simulink model "Instalacion_Cascade"  (R2016b)
settings: Solver=ode23tb  StartTime=0.0  StopTime=2  RelTol=1e-3
libraries: powerlib x50, powerlib_meascontrol x12, simulink x8
settings Model: Creator=acasado  LastModifiedBy=acasado

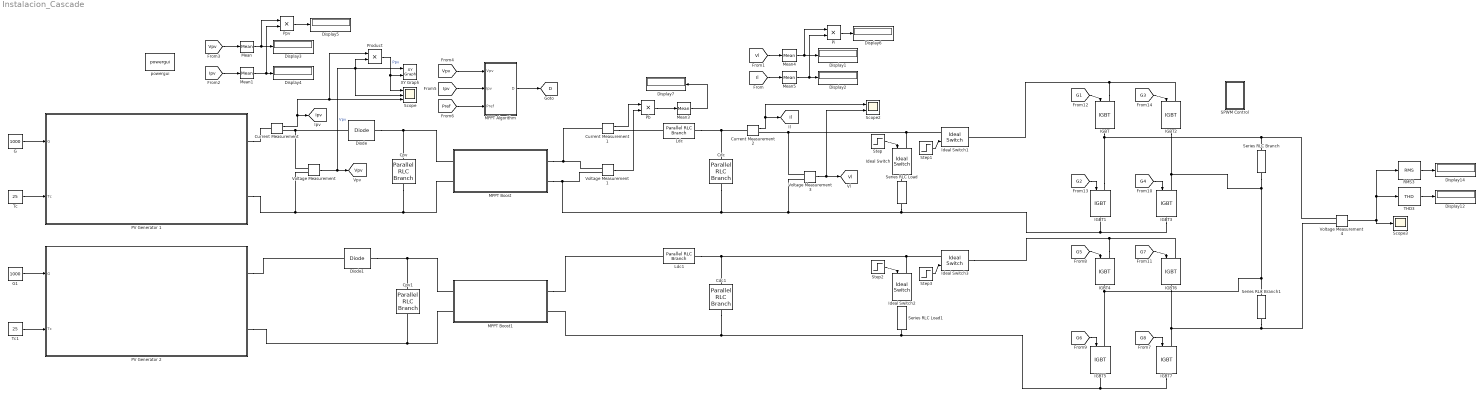
== system Instalacion_Cascade ==
  Cdc : powerlib/Elements/Parallel RLC Branch  LConnTagsString=a  RConnTagsString=__new0  BranchType=C  Resistance=1  Inductance=1e-3  SetiL0=off  InitialCurrent=0  Capacitance=4.7e-5  Setx0=off  InitialVoltage=20  Measurements=None
  Cdc1 : powerlib/Elements/Parallel RLC Branch  LConnTagsString=a  RConnTagsString=__new0  BranchType=C  Resistance=1  Inductance=1e-3  SetiL0=off  InitialCurrent=0  Capacitance=4.7e-5  Setx0=off  InitialVoltage=20  Measurements=None
  Cpv : powerlib/Elements/Parallel RLC Branch  LConnTagsString=a  RConnTagsString=__new0  BranchType=C  Resistance=1  Inductance=1e-3  SetiL0=off  InitialCurrent=0  Capacitance=4.7e-5  Setx0=off  InitialVoltage=0  Measurements=None
  Cpv1 : powerlib/Elements/Parallel RLC Branch  LConnTagsString=a  RConnTagsString=__new0  BranchType=C  Resistance=1  Inductance=1e-3  SetiL0=off  InitialCurrent=0  Capacitance=4.7e-5  Setx0=off  InitialVoltage=0  Measurements=None
  Current Measurement : powerlib/Measurements/Current Measurement  PhasorSimulation=off  OutputType=Complex  PSBequivalent=0
  Current Measurement1 : powerlib/Measurements/Current Measurement  PhasorSimulation=off  OutputType=Complex  PSBequivalent=0
  Current Measurement2 : powerlib/Measurements/Current Measurement  PhasorSimulation=off  OutputType=Complex  PSBequivalent=0
  Diode : powerlib/Power Electronics/Diode  Ron=0.001  Lon=0  Vf=0.8  IC=0  UseSnubber=off  Rs=500  Cs=250e-9  Measurements=off
  Diode1 : powerlib/Power Electronics/Diode  Ron=0.001  Lon=0  Vf=0.8  IC=0  UseSnubber=off  Rs=500  Cs=250e-9  Measurements=off
  Display{1..7,12,14} (9 alike) : Display
      Display5 settings: Decimation=2
      Display6 settings: Decimation=2
      Display7 settings: Decimation=2
  G : Constant  Value=1000
  G1 : Constant  Value=1000
  IGBT{,1..7} (8 alike) : powerlib/Power Electronics/IGBT  Ron=0.001  Lon=0  Vf=1  Tf=1e-6  Tt=2e-6  IC=0  Rs=1e5  Cs=inf  Measurements=off
  Ideal Switch{,1..3} (4 alike) : powerlib/Power Electronics/Ideal Switch  Ron=0.001  Lon=0  IC=0  Rs=1e5  Cs=inf  Measurements=off
  Ldc : powerlib/Elements/Parallel RLC Branch  LConnTagsString=a  RConnTagsString=__new0  BranchType=L  Resistance=1  Inductance=1e-3  SetiL0=off  InitialCurrent=0  Capacitance=1e-6  Setx0=off  InitialVoltage=0  Measurements=None
  Ldc1 : powerlib/Elements/Parallel RLC Branch  LConnTagsString=a  RConnTagsString=__new0  BranchType=L  Resistance=1  Inductance=1e-3  SetiL0=off  InitialCurrent=0  Capacitance=1e-6  Setx0=off  InitialVoltage=0  Measurements=None
  MPPT Algorithm : Subsystem  mask{N=3}
      mask TypeOptions N: 1 | 2 | 3 | 4
  MPPT Boost : Subsystem
      mask Display: image('\\Boole\Proyectos\LI_ROW_2017_SOLAR\BOOST.png')
  MPPT Boost1 : Subsystem
      mask Display: image('\\Boole\Proyectos\LI_ROW_2017_SOLAR\BOOST.png')
  Mean{,1,3..5} (5 alike) : powerlib_meascontrol/Measurements/Mean  Freq=10000  Vinit=0  Ts=0
  PV Generator 1 : Subsystem  mask{G=1000, Tc=25, Pmax=200, Isc=8.21, Voc=32.9, ki=3.18e-3/8.21, kv=-0.123/32.9, Ncs=54, n=1.3417, Rs=0.2172, Rsh=951.9317, Ns=3, Np=3}
      mask prompts: G "G (W/m2)"; Tc "Tc (ºC)"; Pmax "Pmax (W)"; Isc "Isc (A)"; Voc "Voc (V)"; ki "ki (%/º)"; kv "kv (%/º)"; Rs "Rs (ohm)"; Rsh "Rsh (ohm)"
      mask Display: image('\\Boole\Proyectos\LI_ROW_2017_SOLAR\string.jpg')
  PV Generator 2 : Subsystem  mask{G=1000, Tc=25, Pmax=200, Isc=8.21, Voc=32.9, ki=3.18e-3/8.21, kv=-0.123/32.9, Ncs=54, n=1.3417, Rs=0.2172, Rsh=951.9317, Ns=3, Np=3}
      mask prompts: G "G (W/m2)"; Tc "Tc (ºC)"; Pmax "Pmax (W)"; Isc "Isc (A)"; Voc "Voc (V)"; ki "ki (%/º)"; kv "kv (%/º)"; Rs "Rs (ohm)"; Rsh "Rsh (ohm)"
      mask Display: image('\\Boole\Proyectos\LI_ROW_2017_SOLAR\string.jpg')
  Pb : Product
  Pi : Product
  Ppv : Product
  Product : Product
  RMS3 : powerlib_meascontrol/Measurements/RMS  TrueRMS=on  Freq=50  RMSInit=0  Ts=0
  SPWM Control : Subsystem  mask{A=2, fm=3000, fs=50}
  Scope : Scope  NumInputPorts=3
  Scope2 : Scope  NumInputPorts=2
  Scope3 : Scope
  Series RLC Branch : powerlib/Elements/Series RLC Branch  LConnTagsString=__new0  RConnTagsString=__new0  BranchType=R  Resistance=100  Inductance=1e-3  SetiL0=off  InitialCurrent=0  Capacitance=1e-6  Setx0=off  InitialVoltage=0  Measurements=None
  Series RLC Branch1 : powerlib/Elements/Series RLC Branch  LConnTagsString=__new0  RConnTagsString=__new0  BranchType=R  Resistance=100  Inductance=1e-3  SetiL0=off  InitialCurrent=0  Capacitance=1e-6  Setx0=off  InitialVoltage=0  Measurements=None
  Series RLC Load : powerlib/Elements/Series RLC Load  LConnTagsString=a  RConnTagsString=__new0  NominalVoltage=100  NominalFrequency=10000  ActivePower=1000  InductivePower=0  CapacitivePower=0  Setx0=off  InitialVoltage=0  SetiL0=off  InitialCurrent=0  Measurements=None  LoadType=constant Z
  Series RLC Load1 : powerlib/Elements/Series RLC Load  LConnTagsString=a  RConnTagsString=__new0  NominalVoltage=100  NominalFrequency=10000  ActivePower=1000  InductivePower=0  CapacitivePower=0  Setx0=off  InitialVoltage=0  SetiL0=off  InitialCurrent=0  Measurements=None  LoadType=constant Z
  Step : Step  Time=0.02  Before=1  After=0  SampleTime=0
  Step1 : Step  Time=0.02  SampleTime=0
  Step2 : Step  Time=0.02  Before=1  After=0  SampleTime=0
  Step3 : Step  Time=0.02  SampleTime=0
  THD3 : powerlib_meascontrol/Measurements/THD  Freq=50  Ts=0
  Tc : Constant  Value=25
  Tc1 : Constant  Value=25
  Voltage Measurement{,1,3..4} (4 alike) : powerlib/Measurements/Voltage Measurement  PhasorSimulation=off  OutputType=Complex  PSBequivalent=0
  XY Graph : simulink/Sinks/XY Graph  xmin=0  xmax=33  ymin=0  ymax=205  st=-1
  powergui : powerlib/powergui  Priority=1  SimulationMode=Continuous  SolverType=Tustin/Backward Euler (TBE)  SampleTime=50e-6  frequency=60  SPID=off  DisableSnubberDevices=off  DisableRonSwitches=off  DisableVfSwitches=off  SwTol=0  DisplayEquations=off  Interpol=off  ExternalGateDelay=off  methode=off  Ts=10  FunctionMessages=off  echomessages=off  HookPort=off  EnableUseOfTLC=off  x0status=blocks  frequencyindice=0  Pbase=100e6  ErrMax=1e-4  Iterations=50  UnitsV=kV  UnitsW=MW  buscounter=0  RestoreLinks=warning  ResistiveCurrentMeasurement=off  Frange=[0:2:500]  Ylog=off  Xlog=on  ShowGrid=off  save=off  variable=ZData  structure=Bridge  ZoomFFT=on  StartTime=0.2  cycles=5  DisplayStyle=1  fundamental=50  FreqAxis=off  MaxFrequency=1000  frequencyindicesteady=1  RmsSteady=1  display=off
  tag scope: D=global, Il=global, Ipv=global, Vl=global, Vpv=global
  wires:
  Current Measurement/1 -> [Ipv], Scope/3, Product/1
  Voltage Measurement/1 -> [Vpv], Product/2, XY Graph/1, Scope/2  "Vpv"
  Voltage Measurement3/1 -> Scope2/2, [Vl]
  Current Measurement2/1 -> [Il], Scope2/1
  [Vpv] -> Mean/1
  [Ipv] -> Mean1/1
  Mean/1 -> Ppv/1, Display3/1
  Mean1/1 -> Ppv/2, Display4/1
  Product/1 -> Scope/1, XY Graph/2  "Ppv"
  Ppv/1 -> Display5/1
  Voltage Measurement1/1 -> Pb/2
  Current Measurement1/1 -> Pb/1
  Pb/1 -> Mean3/1
  Mean3/1 -> Display7/1
  [Vpv] -> MPPT Algorithm/1(Vpv)
  [Ipv] -> MPPT Algorithm/2(Ipv)
  MPPT Algorithm/1(D) -> [D]
  [Pref] -> MPPT Algorithm/3(Pref)
  [Vl] -> Mean4/1
  Mean4/1 -> Pi/1, Display1/1
  [Il] -> Mean5/1
  Mean5/1 -> Pi/2, Display2/1
  Pi/1 -> Display6/1
  Step/1 -> Ideal Switch/1
  Step1/1 -> Ideal Switch1/1
  G/1 -> PV Generator 1/1(G)
  Tc/1 -> PV Generator 1/2(Tc)
  Voltage Measurement4/1 -> RMS3/1, THD3/1, Scope3/1
  RMS3/1 -> Display14/1
  THD3/1 -> Display12/1
  Step2/1 -> Ideal Switch2/1
  Step3/1 -> Ideal Switch3/1
  [G1] -> IGBT/1
  [G3] -> IGBT2/1
  [G4] -> IGBT3/1
  [G2] -> IGBT1/1
  [G5] -> IGBT4/1
  [G7] -> IGBT6/1
  [G8] -> IGBT7/1
  [G6] -> IGBT5/1
  G1/1 -> PV Generator 2/1(G)
  Tc1/1 -> PV Generator 2/2(Tc)
  connections:
  Voltage Measurement/LConn1 -- Diode/LConn1 -- Current Measurement/RConn1
  Current Measurement1/LConn1 -- Voltage Measurement1/LConn1 -- MPPT Boost/RConn1
  Cdc/LConn1 -- Ldc/RConn1 -- Current Measurement2/LConn1
  Current Measurement1/RConn1 -- Ldc/LConn1
  Cpv/RConn1 -- MPPT Boost/LConn2 -- PV Generator 1/RConn2 -- Voltage Measurement/LConn2
  PV Generator 1/RConn1 -- Current Measurement/LConn1
  Voltage Measurement3/LConn1 -- Ideal Switch/LConn1 -- Ideal Switch1/LConn1 -- Current Measurement2/RConn1
  Ideal Switch/RConn1 -- Series RLC Load/LConn1
  IGBT/LConn1 -- Ideal Switch1/RConn1 -- IGBT2/LConn1
  Cpv/LConn1 -- Diode/RConn1 -- MPPT Boost/LConn1
  IGBT1/LConn1 -- Voltage Measurement4/LConn1 -- Series RLC Branch/LConn1 -- IGBT/RConn1
  IGBT2/RConn1 -- IGBT3/LConn1 -- IGBT5/LConn1 -- IGBT4/RConn1 -- Series RLC Branch1/LConn1 -- Series RLC Branch/RConn1
  MPPT Boost1/RConn1 -- Ldc1/LConn1
  Ldc1/RConn1 -- Cdc1/LConn1 -- Ideal Switch2/LConn1 -- Ideal Switch3/LConn1
  Cdc1/RConn1 -- Series RLC Load1/RConn1 -- IGBT7/RConn1 -- IGBT5/RConn1 -- MPPT Boost1/RConn2
  Series RLC Branch1/RConn1 -- IGBT6/RConn1 -- IGBT7/LConn1 -- Voltage Measurement4/LConn2
  IGBT4/LConn1 -- Ideal Switch3/RConn1 -- IGBT6/LConn1
  Voltage Measurement1/LConn2 -- MPPT Boost/RConn2 -- IGBT3/RConn1 -- IGBT1/RConn1 -- Series RLC Load/RConn1 -- Voltage Measurement3/LConn2 -- Cdc/RConn1
  PV Generator 2/RConn1 -- Diode1/LConn1
  Diode1/RConn1 -- Cpv1/LConn1 -- MPPT Boost1/LConn1
  MPPT Boost1/LConn2 -- Cpv1/RConn1 -- PV Generator 2/RConn2

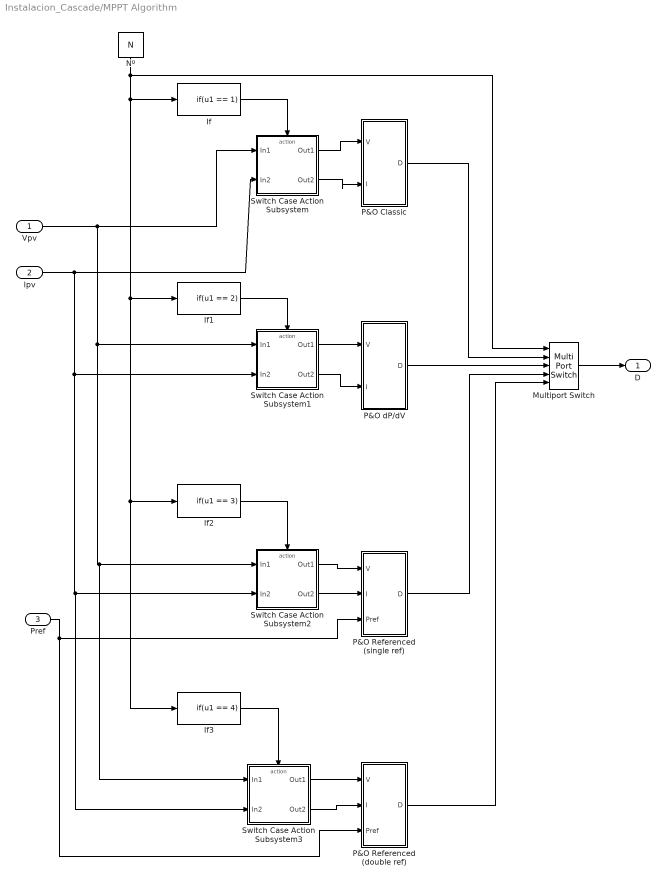
== system Instalacion_Cascade/MPPT Algorithm ==
  Vpv : Inport
  Ipv : Inport  Port=2
  Pref : Inport  Port=3
  If : If  IfExpression=u1 == 1  ShowElse=off
  If1 : If  IfExpression=u1 == 2  ShowElse=off
  If2 : If  IfExpression=u1 == 3  ShowElse=off
  If3 : If  IfExpression=u1 == 4  ShowElse=off
  Multiport Switch : MultiPortSwitch  DataPortOrder=Specify indices  DataPortIndices={1,2,3,4}
  Nº : Constant  Value=N
  P&O Classic : Subsystem
  P&O Referenced (double ref) : Subsystem
  P&O Referenced (single ref) : Subsystem
  P&O dP/dV : Subsystem
  Switch Case Action Subsystem : Subsystem  TreatAsAtomicUnit=on
  Switch Case Action Subsystem1 : Subsystem  TreatAsAtomicUnit=on
  Switch Case Action Subsystem2 : Subsystem  TreatAsAtomicUnit=on
  Switch Case Action Subsystem3 : Subsystem  TreatAsAtomicUnit=on
  D : Outport
  wires:
  Multiport Switch/1 -> D/1
  Pref/1 -> P&O Referenced (single ref)/3(Pref), P&O Referenced (double ref)/3(Pref)
  P&O Classic/1(D) -> Multiport Switch/2
  P&O dP/dV/1(D) -> Multiport Switch/3
  P&O Referenced (single ref)/1(D) -> Multiport Switch/4
  Nº/1 -> Multiport Switch/1, If/1, If3/1, If2/1, If1/1
  Switch Case Action Subsystem/2(Out2) -> P&O Classic/2(I)
  Switch Case Action Subsystem/1(Out1) -> P&O Classic/1(V)
  Switch Case Action Subsystem1/1(Out1) -> P&O dP/dV/1(V)
  Switch Case Action Subsystem1/2(Out2) -> P&O dP/dV/2(I)
  Switch Case Action Subsystem2/2(Out2) -> P&O Referenced (single ref)/2(I)
  Switch Case Action Subsystem2/1(Out1) -> P&O Referenced (single ref)/1(V)
  Vpv/1 -> Switch Case Action Subsystem3/1(In1), Switch Case Action Subsystem2/1(In1), Switch Case Action Subsystem1/1(In1), Switch Case Action Subsystem/1(In1)
  Ipv/1 -> Switch Case Action Subsystem3/2(In2), Switch Case Action Subsystem2/2(In2), Switch Case Action Subsystem1/2(In2), Switch Case Action Subsystem/2(In2)
  If1/1 -> Switch Case Action Subsystem1/Action
  If2/1 -> Switch Case Action Subsystem2/Action
  If/1 -> Switch Case Action Subsystem/Action
  P&O Referenced (double ref)/1(D) -> Multiport Switch/5
  Switch Case Action Subsystem3/1(Out1) -> P&O Referenced (double ref)/1(V)
  Switch Case Action Subsystem3/2(Out2) -> P&O Referenced (double ref)/2(I)
  If3/1 -> Switch Case Action Subsystem3/Action

== system Instalacion_Cascade/MPPT Boost ==
  C : powerlib/Elements/Parallel RLC Branch  LConnTagsString=a  RConnTagsString=__new0  BranchType=C  Resistance=1  Inductance=1e-3  SetiL0=off  InitialCurrent=0  Capacitance=3.2e-4  Setx0=off  InitialVoltage=20  Measurements=None
  Diode : powerlib/Power Electronics/Diode  Ron=0.001  Lon=0  Vf=0.8  IC=0  UseSnubber=off  Rs=500  Cs=250e-9  Measurements=off
  L : powerlib/Elements/Parallel RLC Branch  LConnTagsString=a  RConnTagsString=__new0  BranchType=L  Resistance=1  Inductance=1e-3  SetiL0=off  InitialCurrent=0  Capacitance=1e-6  Setx0=off  InitialVoltage=0  Measurements=None
  Mosfet : powerlib/Power Electronics/Mosfet  Ron=0.1  Lon=0  Rd=0.01  Vfd=0  IC=0  Rs=1e5  Cs=inf  Measurements=off
  Conn1 : PMIOPort  Port=1  Side=Left
  Conn3 : PMIOPort  Port=2  Side=Left
  Conn2 : PMIOPort  Port=3  Side=Right
  Conn4 : PMIOPort  Port=4  Side=Right
  wires:
  [D] -> Mosfet/1
  connections:
  Diode/RConn1 -- C/LConn1 -- Conn2/RConn1
  L/LConn1 -- Conn1/RConn1
  Mosfet/LConn1 -- Diode/LConn1 -- L/RConn1
  C/RConn1 -- Conn4/RConn1 -- Conn3/RConn1 -- Mosfet/RConn1

== system Instalacion_Cascade/MPPT Boost1 ==
  C : powerlib/Elements/Parallel RLC Branch  LConnTagsString=a  RConnTagsString=__new0  BranchType=C  Resistance=1  Inductance=1e-3  SetiL0=off  InitialCurrent=0  Capacitance=3.2e-4  Setx0=off  InitialVoltage=20  Measurements=None
  Diode : powerlib/Power Electronics/Diode  Ron=0.001  Lon=0  Vf=0.8  IC=0  UseSnubber=off  Rs=500  Cs=250e-9  Measurements=off
  L : powerlib/Elements/Parallel RLC Branch  LConnTagsString=a  RConnTagsString=__new0  BranchType=L  Resistance=1  Inductance=1e-3  SetiL0=off  InitialCurrent=0  Capacitance=1e-6  Setx0=off  InitialVoltage=0  Measurements=None
  Mosfet : powerlib/Power Electronics/Mosfet  Ron=0.1  Lon=0  Rd=0.01  Vfd=0  IC=0  Rs=1e5  Cs=inf  Measurements=off
  Conn1 : PMIOPort  Port=1  Side=Left
  Conn3 : PMIOPort  Port=2  Side=Left
  Conn2 : PMIOPort  Port=3  Side=Right
  Conn4 : PMIOPort  Port=4  Side=Right
  wires:
  [D] -> Mosfet/1
  connections:
  Mosfet/RConn1 -- Conn3/RConn1 -- Conn4/RConn1 -- C/RConn1
  L/RConn1 -- Diode/LConn1 -- Mosfet/LConn1
  L/LConn1 -- Conn1/RConn1
  Conn2/RConn1 -- C/LConn1 -- Diode/RConn1

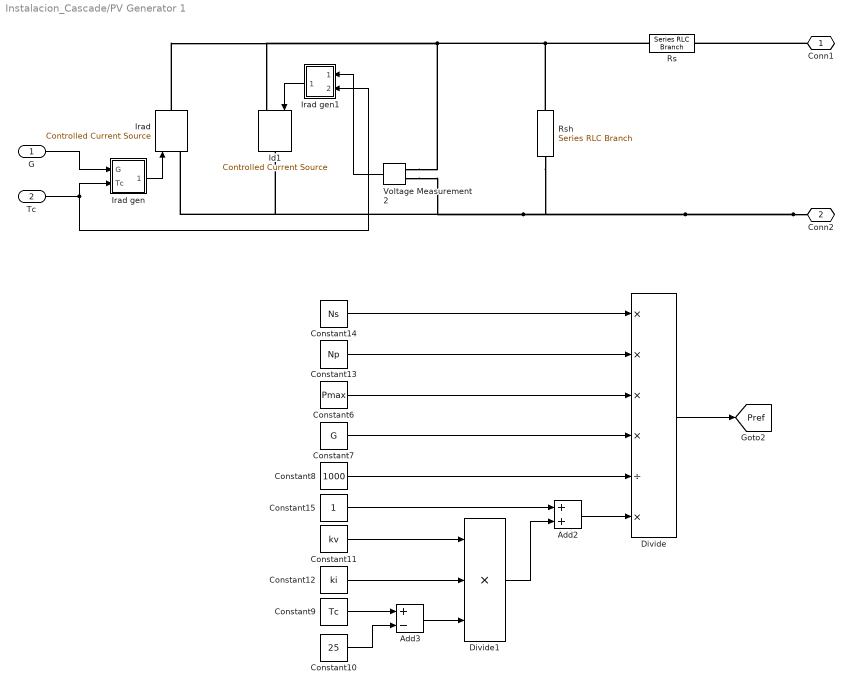
== system Instalacion_Cascade/PV Generator 1 ==
  G : Inport
  Tc : Inport  Port=2
  Add2 : Sum
  Add3 : Sum  Inputs=+-
  Constant10 : Constant  Value=25
  Constant11 : Constant  Value=kv
  Constant12 : Constant  Value=ki
  Constant13 : Constant  Value=Np
  Constant14 : Constant  Value=Ns
  Constant15 : Constant
  Constant6 : Constant  Value=Pmax
  Constant7 : Constant  Value=G
  Constant8 : Constant  Value=1000
  Constant9 : Constant  Value=Tc
  Divide : Product  Inputs=****/*
  Divide1 : Product  Inputs=***
  Id1 : powerlib/Electrical Sources/Controlled Current Source  Initialize=on  Source_Type=DC  Amplitude=0  Phase=0  Frequency=0  Measurements=None
  Irad : powerlib/Electrical Sources/Controlled Current Source  Initialize=off  Source_Type=DC  Amplitude=1  Phase=0  Frequency=0  Measurements=None
  Irad gen : Subsystem  mask{G=G, Tc=Tc, Isc=Isc, ki=ki, Np=Np}
  Irad gen1 : Subsystem  mask{n=n, Isc=Isc, Voc=Voc, ki=ki*Isc, kv=kv*Voc, Tc=Tc, Ncs=Ncs, Ns=Ns, Np=Np}
  Rs : powerlib/Elements/Series RLC Branch  LConnTagsString=__new0  RConnTagsString=__new0  BranchType=R  Resistance=Rs*Ns/Np  Inductance=1e-3  SetiL0=off  InitialCurrent=0  Capacitance=1e-6  Setx0=off  InitialVoltage=0  Measurements=None
  Rsh : powerlib/Elements/Series RLC Branch  LConnTagsString=__new0  RConnTagsString=__new0  BranchType=R  Resistance=Rsh*Ns/Np  Inductance=1e-3  SetiL0=off  InitialCurrent=0  Capacitance=1e-6  Setx0=off  InitialVoltage=0  Measurements=None
  Voltage Measurement2 : powerlib/Measurements/Voltage Measurement  PhasorSimulation=off  OutputType=Complex  PSBequivalent=0
  Conn1 : PMIOPort  Port=1  Side=Right
  Conn2 : PMIOPort  Port=2  Side=Right
  tag scope: Pref=global
  wires:
  Irad gen1/1(Id) -> Id1/1
  Voltage Measurement2/1 -> Irad gen1/1(Vd)
  Irad gen/1(Irad) -> Irad/1
  G/1 -> Irad gen/1(G)
  Tc/1 -> Irad gen1/2(Tc), Irad gen/2(Tc)
  Constant14/1 -> Divide/1
  Constant13/1 -> Divide/2
  Constant6/1 -> Divide/3
  Constant7/1 -> Divide/4
  Constant8/1 -> Divide/5
  Constant15/1 -> Add2/1
  Add2/1 -> Divide/6
  Divide1/1 -> Add2/2
  Constant9/1 -> Add3/1
  Constant10/1 -> Add3/2
  Add3/1 -> Divide1/3
  Constant11/1 -> Divide1/1
  Constant12/1 -> Divide1/2
  Divide/1 -> [Pref]
  connections:
  Conn2/RConn1 -- Id1/RConn1 -- Irad/LConn1 -- Voltage Measurement2/LConn2 -- Rsh/RConn1
  Rsh/LConn1 -- Rs/LConn1 -- Voltage Measurement2/LConn1 -- Id1/LConn1 -- Irad/RConn1
  Conn1/RConn1 -- Rs/RConn1

== system Instalacion_Cascade/PV Generator 2 ==
  G : Inport
  Tc : Inport  Port=2
  Id1 : powerlib/Electrical Sources/Controlled Current Source  Initialize=on  Source_Type=DC  Amplitude=0  Phase=0  Frequency=0  Measurements=None
  Irad : powerlib/Electrical Sources/Controlled Current Source  Initialize=off  Source_Type=DC  Amplitude=1  Phase=0  Frequency=0  Measurements=None
  Irad gen : Subsystem  mask{G=G, Tc=Tc, Isc=Isc, ki=ki, Np=Np}
  Irad gen1 : Subsystem  mask{n=n, Isc=Isc, Voc=Voc, ki=ki*Isc, kv=kv*Voc, Tc=Tc, Ncs=Ncs, Ns=Ns, Np=Np}
  Rs : powerlib/Elements/Series RLC Branch  LConnTagsString=__new0  RConnTagsString=__new0  BranchType=R  Resistance=Rs*Ns/Np  Inductance=1e-3  SetiL0=off  InitialCurrent=0  Capacitance=1e-6  Setx0=off  InitialVoltage=0  Measurements=None
  Rsh : powerlib/Elements/Series RLC Branch  LConnTagsString=__new0  RConnTagsString=__new0  BranchType=R  Resistance=Rsh*Ns/Np  Inductance=1e-3  SetiL0=off  InitialCurrent=0  Capacitance=1e-6  Setx0=off  InitialVoltage=0  Measurements=None
  Voltage Measurement2 : powerlib/Measurements/Voltage Measurement  PhasorSimulation=off  OutputType=Complex  PSBequivalent=0
  Conn1 : PMIOPort  Port=1  Side=Right
  Conn2 : PMIOPort  Port=2  Side=Right
  wires:
  Tc/1 -> Irad gen/2(Tc), Irad gen1/2(Tc)
  G/1 -> Irad gen/1(G)
  Irad gen/1(Irad) -> Irad/1
  Voltage Measurement2/1 -> Irad gen1/1(Vd)
  Irad gen1/1(Id) -> Id1/1
  connections:
  Conn1/RConn1 -- Rs/RConn1
  Irad/RConn1 -- Id1/LConn1 -- Voltage Measurement2/LConn1 -- Rs/LConn1 -- Rsh/LConn1
  Rsh/RConn1 -- Voltage Measurement2/LConn2 -- Irad/LConn1 -- Id1/RConn1 -- Conn2/RConn1

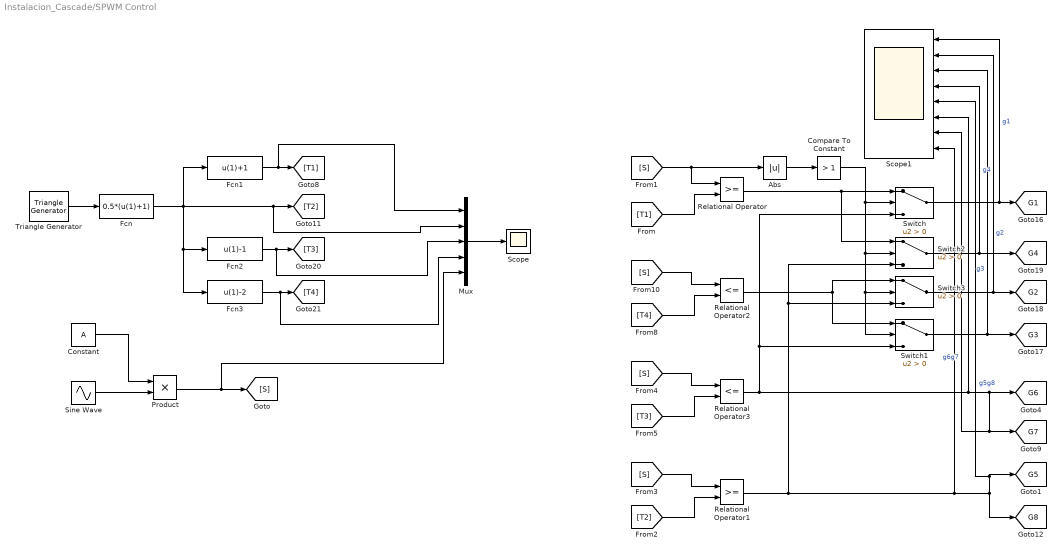
== system Instalacion_Cascade/SPWM Control ==
  Abs : Abs
  Compare To Constant : simulink/Logic and Bit Operations/Compare To Constant  relop=>  const=1  OutDataTypeStr=boolean
  Constant : Constant  Value=A
  Fcn : Fcn  Expr=0.5*(u(1)+1)
  Fcn1 : Fcn  Expr=u(1)+1
  Fcn2 : Fcn  Expr=u(1)-1
  Fcn3 : Fcn  Expr=u(1)-2
  Mux : Mux  Inputs=5
  Product : Product
  Relational Operator : RelationalOperator  OutDataTypeStr=boolean  RndMeth=Simplest
  Relational Operator1 : RelationalOperator  OutDataTypeStr=boolean  RndMeth=Simplest
  Relational Operator2 : RelationalOperator  Operator=<=  OutDataTypeStr=boolean  RndMeth=Simplest
  Relational Operator3 : RelationalOperator  Operator=<=  OutDataTypeStr=boolean  RndMeth=Simplest
  Scope : Scope
  Scope1 : Scope  NumInputPorts=8
  Sine Wave : Sin  Frequency=fs*2*pi  SampleTime=0
  Switch{,1..3} (4 alike) : Switch  Criteria=u2 > Threshold
  Triangle Generator : powerlib_meascontrol/Pulse & Signal Generators/Triangle Generator  Freq=fm  Phase=90  Ts=0
  tag scope: G1=global, G2=global, G3=global, G4=global, G5=global, G6=global, G7=global, G8=global
  wires:
  Sine Wave/1 -> Product/2
  Constant/1 -> Product/1
  Product/1 -> Mux/5, [S]
  Fcn/1 -> Mux/2, [T2], Fcn2/1, Fcn3/1, Fcn1/1
  Fcn1/1 -> Mux/1, [T1]
  Fcn2/1 -> Mux/3, [T3]
  Fcn3/1 -> Mux/4, [T4]
  Triangle Generator/1 -> Fcn/1
  Mux/1 -> Scope/1
  [S] -> Abs/1, Relational Operator/1
  [T1] -> Relational Operator/2
  [S] -> Relational Operator2/1
  [T4] -> Relational Operator2/2
  [S] -> Relational Operator1/1
  [T2] -> Relational Operator1/2
  [S] -> Relational Operator3/1
  [T3] -> Relational Operator3/2
  Switch/1 -> Scope1/1, [G1]  "g1"
  Relational Operator/1 -> Switch2/1, Switch/1
  Abs/1 -> Compare To Constant/1
  Compare To Constant/1 -> Switch2/2, Switch3/2, Switch1/2, Switch/2
  Relational Operator1/1 -> Switch3/3, Switch2/3, Scope1/8, Scope1/5, [G5], [G8]  "g5g8"
  Switch1/1 -> Scope1/3, [G3]  "g3"
  Relational Operator2/1 -> Switch3/1, Switch1/1
  Relational Operator3/1 -> Switch1/3, Switch/3, Scope1/6, Scope1/7, [G7], [G6]  "g6g7"
  Switch2/1 -> Scope1/4, [G4]  "g4"
  Switch3/1 -> Scope1/2, [G2]  "g2"

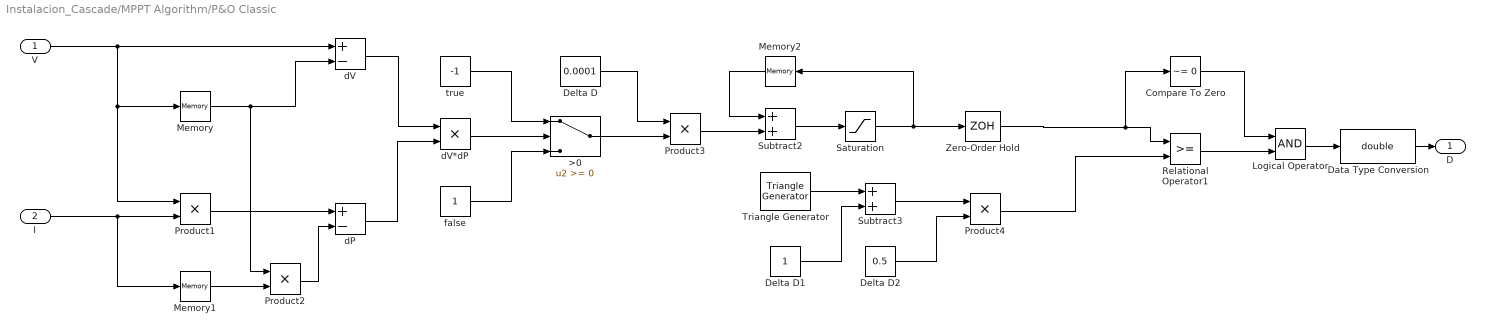
== system Instalacion_Cascade/MPPT Algorithm/P&O Classic ==
  V : Inport
  I : Inport  Port=2
  >0 : Switch  ZeroCross=off
  Compare To Zero : simulink/Logic and Bit Operations/Compare To Zero  relop=~=  OutDataTypeStr=boolean
  Data Type Conversion : DataTypeConversion  OutDataTypeStr=double
  Delta D : Constant  Value=0.0001
  Delta D1 : Constant
  Delta D2 : Constant  Value=0.5
  Logical Operator : Logic  AllPortsSameDT=off  OutDataTypeStr=boolean
  Memory : Memory
  Memory1 : Memory  X0=8.21
  Memory2 : Memory  X0=0.5
  Product{1..4} (4 alike) : Product
  Relational Operator1 : RelationalOperator  OutDataTypeStr=boolean  RndMeth=Simplest
  Saturation : Saturate  UpperLimit=1  LowerLimit=0
  Subtract2 : Sum
  Subtract3 : Sum
  Triangle Generator : powerlib_meascontrol/Pulse & Signal Generators/Triangle Generator  Freq=10000  Phase=0  Ts=0
  Zero-Order Hold : ZeroOrderHold  SampleTime=1/5000
  dP : Sum  Inputs=+-
  dV : Sum  Inputs=+-
  dV*dP : Product
  false : Constant
  true : Constant  Value=-1
  D : Outport
  wires:
  false/1 -> >0/3
  dP/1 -> dV*dP/2
  true/1 -> >0/1
  >0/1 -> Product3/2
  Delta D/1 -> Product3/1
  Memory/1 -> Product2/1, dV/2
  Subtract2/1 -> Saturation/1
  dV/1 -> dV*dP/1
  dV*dP/1 -> >0/2
  Triangle Generator/1 -> Subtract3/1
  Delta D1/1 -> Subtract3/2
  Product4/1 -> Relational Operator1/2
  Subtract3/1 -> Product4/1
  Product3/1 -> Subtract2/2
  Memory2/1 -> Subtract2/1
  Delta D2/1 -> Product4/2
  V/1 -> dV/1, Memory/1, Product1/1
  Saturation/1 -> Memory2/1, Zero-Order Hold/1
  I/1 -> Memory1/1, Product1/2
  Product1/1 -> dP/1
  Zero-Order Hold/1 -> Compare To Zero/1, Relational Operator1/1
  Memory1/1 -> Product2/2
  Product2/1 -> dP/2
  Compare To Zero/1 -> Logical Operator/1
  Relational Operator1/1 -> Logical Operator/2
  Logical Operator/1 -> Data Type Conversion/1
  Data Type Conversion/1 -> D/1

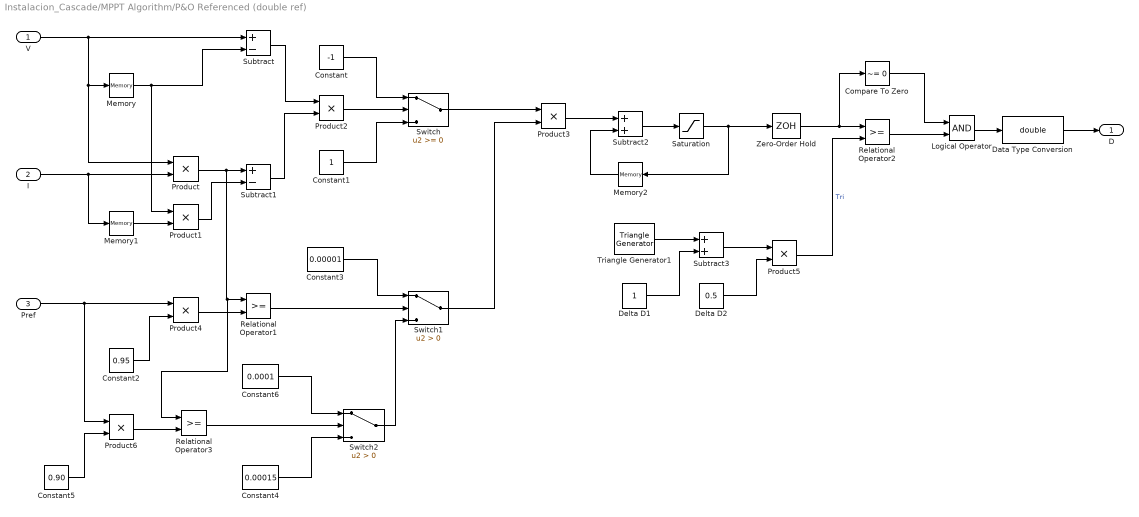
== system Instalacion_Cascade/MPPT Algorithm/P&O Referenced (double ref) ==
  V : Inport
  I : Inport  Port=2
  Pref : Inport  Port=3
  Compare To Zero : simulink/Logic and Bit Operations/Compare To Zero  relop=~=  OutDataTypeStr=boolean
  Constant : Constant  Value=-1
  Constant1 : Constant
  Constant2 : Constant  Value=0.95
  Constant3 : Constant  Value=0.00001
  Constant4 : Constant  Value=0.00015
  Constant5 : Constant  Value=0.90
  Constant6 : Constant  Value=0.0001
  Data Type Conversion : DataTypeConversion  OutDataTypeStr=double
  Delta D1 : Constant
  Delta D2 : Constant  Value=0.5
  Logical Operator : Logic  AllPortsSameDT=off  OutDataTypeStr=boolean
  Memory : Memory
  Memory1 : Memory  X0=8.21
  Memory2 : Memory  X0=0.5
  Product{,1..6} (7 alike) : Product
  Relational Operator1 : RelationalOperator  OutDataTypeStr=boolean  RndMeth=Simplest
  Relational Operator2 : RelationalOperator  OutDataTypeStr=boolean  RndMeth=Simplest
  Relational Operator3 : RelationalOperator  OutDataTypeStr=boolean  RndMeth=Simplest
  Saturation : Saturate  UpperLimit=1  LowerLimit=0
  Subtract : Sum  Inputs=+-
  Subtract1 : Sum  Inputs=+-
  Subtract2 : Sum
  Subtract3 : Sum
  Switch : Switch
  Switch1 : Switch  Criteria=u2 > Threshold
  Switch2 : Switch  Criteria=u2 > Threshold
  Triangle Generator1 : powerlib_meascontrol/Pulse & Signal Generators/Triangle Generator  Freq=10000  Phase=0  Ts=0
  Zero-Order Hold : ZeroOrderHold  SampleTime=1/5000
  D : Outport
  wires:
  Pref/1 -> Product6/1, Product4/1
  Data Type Conversion/1 -> D/1
  Zero-Order Hold/1 -> Compare To Zero/1, Relational Operator2/1
  Logical Operator/1 -> Data Type Conversion/1
  Relational Operator2/1 -> Logical Operator/2
  Compare To Zero/1 -> Logical Operator/1
  Product5/1 -> Relational Operator2/2  "Tri"
  Delta D2/1 -> Product5/2
  Subtract3/1 -> Product5/1
  Delta D1/1 -> Subtract3/2
  Triangle Generator1/1 -> Subtract3/1
  Switch1/1 -> Product3/2
  Constant3/1 -> Switch1/1
  Relational Operator1/1 -> Switch1/2
  Product4/1 -> Relational Operator1/2
  Constant2/1 -> Product4/2
  Switch/1 -> Product3/1
  Constant1/1 -> Switch/3
  Subtract1/1 -> Product2/2
  Constant/1 -> Switch/1
  V/1 -> Product/1, Memory/1, Subtract/1
  Memory/1 -> Product1/1, Subtract/2
  Memory2/1 -> Subtract2/2
  Product3/1 -> Subtract2/1
  I/1 -> Memory1/1, Product/2
  Subtract2/1 -> Saturation/1
  Memory1/1 -> Product1/2
  Product/1 -> Subtract1/1, Relational Operator3/1, Relational Operator1/1
  Product1/1 -> Subtract1/2
  Subtract/1 -> Product2/1
  Product2/1 -> Switch/2
  Saturation/1 -> Memory2/1, Zero-Order Hold/1
  Relational Operator3/1 -> Switch2/2
  Product6/1 -> Relational Operator3/2
  Constant5/1 -> Product6/2
  Constant6/1 -> Switch2/1
  Constant4/1 -> Switch2/3
  Switch2/1 -> Switch1/3

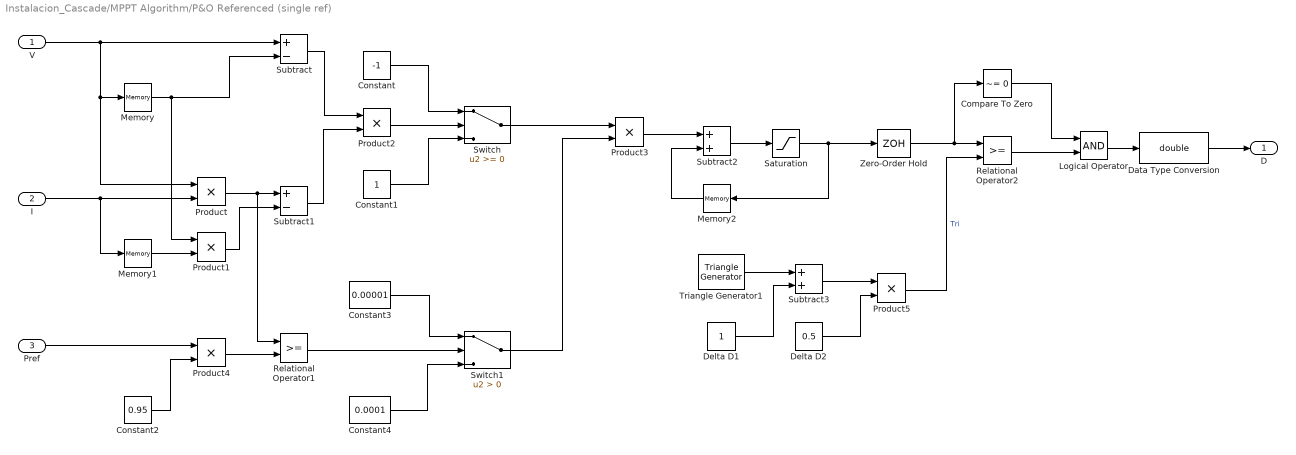
== system Instalacion_Cascade/MPPT Algorithm/P&O Referenced (single ref) ==
  V : Inport
  I : Inport  Port=2
  Pref : Inport  Port=3
  Compare To Zero : simulink/Logic and Bit Operations/Compare To Zero  relop=~=  OutDataTypeStr=boolean
  Constant : Constant  Value=-1
  Constant1 : Constant
  Constant2 : Constant  Value=0.95
  Constant3 : Constant  Value=0.00001
  Constant4 : Constant  Value=0.0001
  Data Type Conversion : DataTypeConversion  OutDataTypeStr=double
  Delta D1 : Constant
  Delta D2 : Constant  Value=0.5
  Logical Operator : Logic  AllPortsSameDT=off  OutDataTypeStr=boolean
  Memory : Memory
  Memory1 : Memory  X0=8.21
  Memory2 : Memory  X0=0.5
  Product{,1..5} (6 alike) : Product
  Relational Operator1 : RelationalOperator  OutDataTypeStr=boolean  RndMeth=Simplest
  Relational Operator2 : RelationalOperator  OutDataTypeStr=boolean  RndMeth=Simplest
  Saturation : Saturate  UpperLimit=1  LowerLimit=0
  Subtract : Sum  Inputs=+-
  Subtract1 : Sum  Inputs=+-
  Subtract2 : Sum
  Subtract3 : Sum
  Switch : Switch
  Switch1 : Switch  Criteria=u2 > Threshold
  Triangle Generator1 : powerlib_meascontrol/Pulse & Signal Generators/Triangle Generator  Freq=10000  Phase=0  Ts=0
  Zero-Order Hold : ZeroOrderHold  SampleTime=1/5000
  D : Outport
  wires:
  Saturation/1 -> Zero-Order Hold/1, Memory2/1
  Product2/1 -> Switch/2
  Subtract/1 -> Product2/1
  Product1/1 -> Subtract1/2
  Product/1 -> Relational Operator1/1, Subtract1/1
  Memory1/1 -> Product1/2
  Subtract2/1 -> Saturation/1
  I/1 -> Product/2, Memory1/1
  Product3/1 -> Subtract2/1
  Memory2/1 -> Subtract2/2
  Memory/1 -> Subtract/2, Product1/1
  V/1 -> Subtract/1, Memory/1, Product/1
  Constant/1 -> Switch/1
  Subtract1/1 -> Product2/2
  Constant1/1 -> Switch/3
  Switch/1 -> Product3/1
  Constant2/1 -> Product4/2
  Product4/1 -> Relational Operator1/2
  Relational Operator1/1 -> Switch1/2
  Constant3/1 -> Switch1/1
  Constant4/1 -> Switch1/3
  Switch1/1 -> Product3/2
  Triangle Generator1/1 -> Subtract3/1
  Delta D1/1 -> Subtract3/2
  Subtract3/1 -> Product5/1
  Delta D2/1 -> Product5/2
  Product5/1 -> Relational Operator2/2  "Tri"
  Compare To Zero/1 -> Logical Operator/1
  Relational Operator2/1 -> Logical Operator/2
  Logical Operator/1 -> Data Type Conversion/1
  Zero-Order Hold/1 -> Relational Operator2/1, Compare To Zero/1
  Data Type Conversion/1 -> D/1
  Pref/1 -> Product4/1

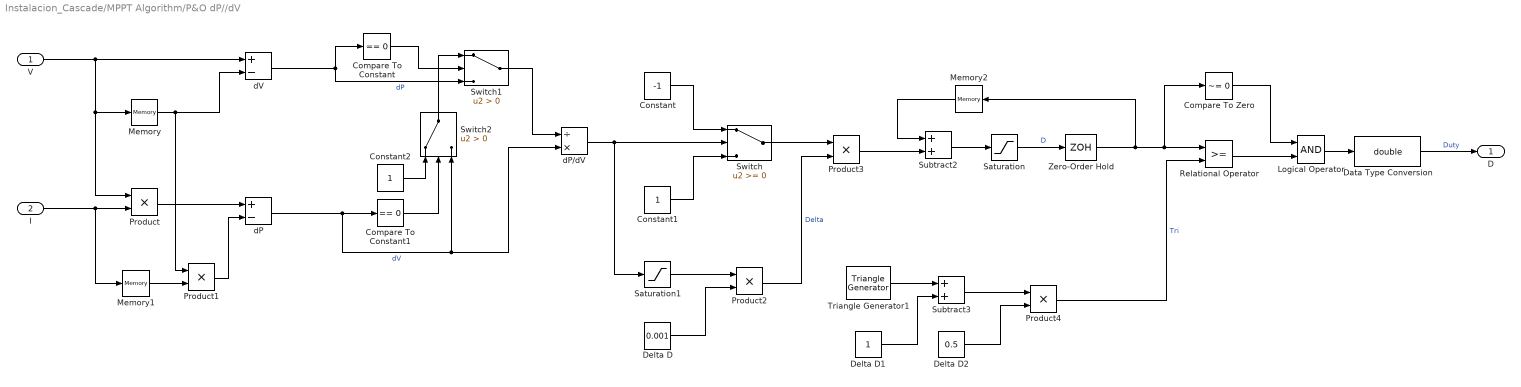
== system Instalacion_Cascade/MPPT Algorithm/P&O dP//dV ==
  V : Inport
  I : Inport  Port=2
  Compare To Constant : simulink/Logic and Bit Operations/Compare To Constant  relop===  const=0  OutDataTypeStr=boolean  ZeroCross=off
  Compare To Constant1 : simulink/Logic and Bit Operations/Compare To Constant  relop===  const=0  OutDataTypeStr=boolean  ZeroCross=off
  Compare To Zero : simulink/Logic and Bit Operations/Compare To Zero  relop=~=  OutDataTypeStr=boolean
  Constant : Constant  Value=-1
  Constant1 : Constant
  Constant2 : Constant
  Data Type Conversion : DataTypeConversion  OutDataTypeStr=double
  Delta D : Constant  Value=0.001
  Delta D1 : Constant
  Delta D2 : Constant  Value=0.5
  Logical Operator : Logic  AllPortsSameDT=off  OutDataTypeStr=boolean
  Memory : Memory
  Memory1 : Memory  X0=8.21
  Memory2 : Memory  X0=0.5
  Product{,1..4} (5 alike) : Product
  Relational Operator : RelationalOperator  OutDataTypeStr=boolean  RndMeth=Simplest
  Saturation : Saturate  UpperLimit=1  LowerLimit=0  ZeroCross=off
  Saturation1 : Saturate  UpperLimit=1  LowerLimit=0.1  ZeroCross=off
  Subtract2 : Sum
  Subtract3 : Sum
  Switch : Switch  ZeroCross=off
  Switch1 : Switch  Criteria=u2 > Threshold  ZeroCross=off
  Switch2 : Switch  Criteria=u2 > Threshold  ZeroCross=off
  Triangle Generator1 : powerlib_meascontrol/Pulse & Signal Generators/Triangle Generator  Freq=10000  Phase=0  Ts=0
  Zero-Order Hold : ZeroOrderHold  SampleTime=1/5000
  dP : Sum  Inputs=+-
  dP/dV : Product  Inputs=/*
  dV : Sum  Inputs=+-
  D : Outport
  wires:
  Saturation/1 -> Zero-Order Hold/1  "D"
  dP/dV/1 -> Saturation1/1, Switch/2
  Product/1 -> dP/1
  Subtract2/1 -> Saturation/1
  I/1 -> Memory1/1, Product/2
  Memory/1 -> dV/2, Product1/1
  Switch/1 -> Product3/1
  V/1 -> dV/1, Memory/1, Product/1
  Constant/1 -> Switch/1
  Constant1/1 -> Switch/3
  Product4/1 -> Relational Operator/2  "Tri"
  Saturation1/1 -> Product2/1
  Delta D/1 -> Product2/2
  Product2/1 -> Product3/2  "Delta"
  Triangle Generator1/1 -> Subtract3/1
  Delta D1/1 -> Subtract3/2
  Subtract3/1 -> Product4/1
  Delta D2/1 -> Product4/2
  Product3/1 -> Subtract2/2
  Memory2/1 -> Subtract2/1
  dV/1 -> Compare To Constant/1, Switch1/3  "dP"
  Switch1/1 -> dP/dV/1
  dP/1 -> Compare To Constant1/1, Switch2/3, dP/dV/2  "dV"
  Compare To Zero/1 -> Logical Operator/1
  Relational Operator/1 -> Logical Operator/2
  Logical Operator/1 -> Data Type Conversion/1
  Data Type Conversion/1 -> D/1  "Duty"
  Zero-Order Hold/1 -> Memory2/1, Compare To Zero/1, Relational Operator/1
  Product1/1 -> dP/2
  Memory1/1 -> Product1/2
  Compare To Constant/1 -> Switch1/2
  Compare To Constant1/1 -> Switch2/2
  Constant2/1 -> Switch2/1
  Switch2/1 -> Switch1/1

== system Instalacion_Cascade/MPPT Algorithm/Switch Case Action Subsystem ==
  In1 : Inport
  In2 : Inport  Port=2
  Action Port : ActionPort  ActionType=then
  Out1 : Outport
  Out2 : Outport  Port=2
  wires:
  In1/1 -> Out1/1
  In2/1 -> Out2/1

== system Instalacion_Cascade/MPPT Algorithm/Switch Case Action Subsystem1 ==
  In1 : Inport
  In2 : Inport  Port=2
  Action Port : ActionPort  ActionType=then
  Out1 : Outport
  Out2 : Outport  Port=2
  wires:
  In2/1 -> Out2/1
  In1/1 -> Out1/1

== system Instalacion_Cascade/MPPT Algorithm/Switch Case Action Subsystem2 ==
  In1 : Inport
  In2 : Inport  Port=2
  Action Port : ActionPort  ActionType=then
  Out1 : Outport
  Out2 : Outport  Port=2
  wires:
  In1/1 -> Out1/1
  In2/1 -> Out2/1

== system Instalacion_Cascade/MPPT Algorithm/Switch Case Action Subsystem3 ==
  In1 : Inport
  In2 : Inport  Port=2
  Action Port : ActionPort  ActionType=then
  Out1 : Outport
  Out2 : Outport  Port=2
  wires:
  In2/1 -> Out2/1
  In1/1 -> Out1/1

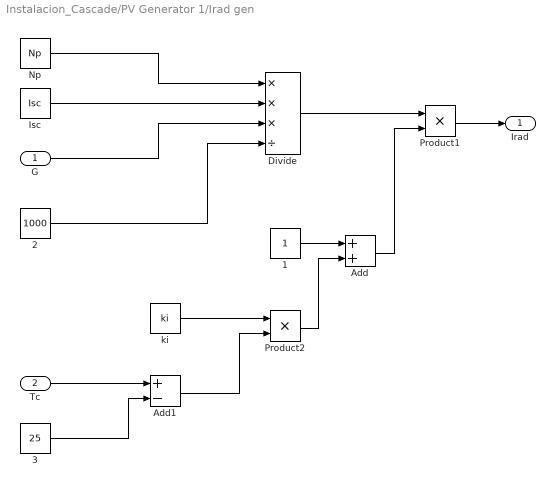
== system Instalacion_Cascade/PV Generator 1/Irad gen ==
  G : Inport
  Tc : Inport  Port=2
  1 : Constant
  2 : Constant  Value=1000
  3 : Constant  Value=25
  Add : Sum
  Add1 : Sum  Inputs=+-
  Divide : Product  Inputs=***/
  Isc : Constant  Value=Isc
  Np : Constant  Value=Np
  Product1 : Product
  Product2 : Product
  ki : Constant  Value=ki
  Irad : Outport
  wires:
  Product1/1 -> Irad/1
  3/1 -> Add1/2
  Add1/1 -> Product2/2
  Tc/1 -> Add1/1
  Product2/1 -> Add/2
  Add/1 -> Product1/2
  1/1 -> Add/1
  ki/1 -> Product2/1
  Divide/1 -> Product1/1
  Np/1 -> Divide/1
  Isc/1 -> Divide/2
  G/1 -> Divide/3
  2/1 -> Divide/4

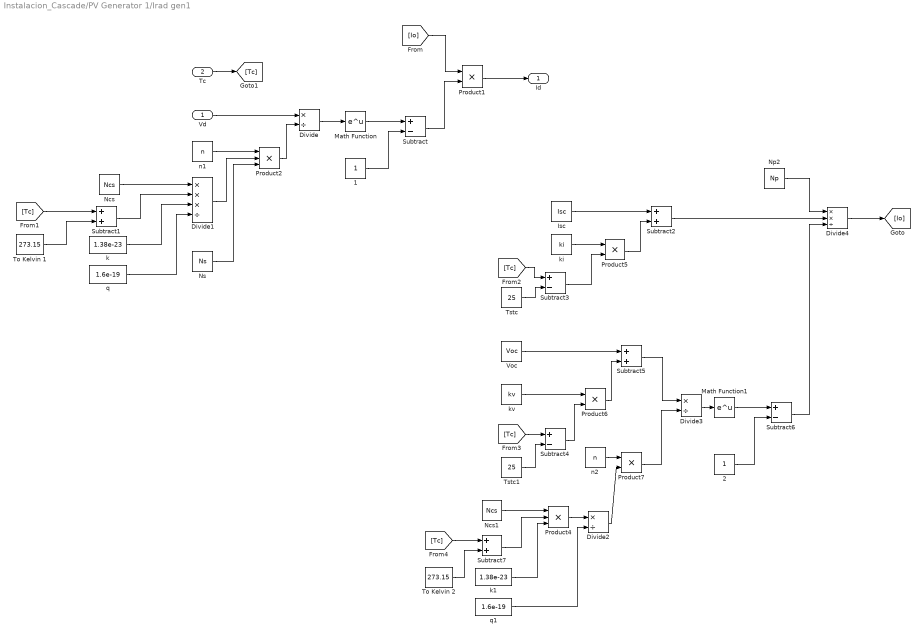
== system Instalacion_Cascade/PV Generator 1/Irad gen1 ==
  Vd : Inport
  Tc : Inport  Port=2
  1 : Constant
  2 : Constant
  Divide : Product  Inputs=*/
  Divide1 : Product  Inputs=***/
  Divide2 : Product  Inputs=*/
  Divide3 : Product  Inputs=*/
  Divide4 : Product  Inputs=**/
  Isc : Constant  Value=Isc
  Math Function : Math  SaturateOnIntegerOverflow=on
  Math Function1 : Math  SaturateOnIntegerOverflow=on
  Ncs : Constant  Value=Ncs
  Ncs1 : Constant  Value=Ncs
  Np2 : Constant  Value=Np
  Ns : Constant  Value=Ns
  Product{1,5..7} (4 alike) : Product
  Product2 : Product  Inputs=3
  Product4 : Product  Inputs=3
  Subtract{,3..4,6} (4 alike) : Sum  Inputs=+-
  Subtract{1..2,5,7} (4 alike) : Sum
  To Kelvin 1 : Constant  Value=273.15
  To Kelvin 2 : Constant  Value=273.15
  Tstc : Constant  Value=25
  Tstc1 : Constant  Value=25
  Voc : Constant  Value=Voc
  k : Constant  Value=1.38e-23
  k1 : Constant  Value=1.38e-23
  ki : Constant  Value=ki
  kv : Constant  Value=kv
  n1 : Constant  Value=n
  n2 : Constant  Value=n
  q : Constant  Value=1.6e-19
  q1 : Constant  Value=1.6e-19
  Id : Outport
  wires:
  To Kelvin 2/1 -> Subtract7/2
  Subtract7/1 -> Product4/2
  [Tc] -> Subtract7/1
  To Kelvin 1/1 -> Subtract1/2
  [Tc] -> Subtract1/1
  Subtract1/1 -> Divide1/2
  q/1 -> Divide1/4
  k/1 -> Divide1/3
  Ncs/1 -> Divide1/1
  Divide1/1 -> Product2/2
  n1/1 -> Product2/1
  Product2/1 -> Divide/2
  Divide4/1 -> [Io]
  Math Function1/1 -> Subtract6/1
  2/1 -> Subtract6/2
  Divide3/1 -> Math Function1/1
  Product6/1 -> Subtract5/2
  n2/1 -> Product7/1
  Subtract4/1 -> Product6/2
  kv/1 -> Product6/1
  Tstc1/1 -> Subtract4/2
  [Tc] -> Subtract4/1
  Subtract3/1 -> Product5/2
  Tstc/1 -> Subtract3/2
  [Tc] -> Subtract3/1
  Product5/1 -> Subtract2/2
  ki/1 -> Product5/1
  Divide2/1 -> Product7/2
  q1/1 -> Divide2/2
  Product4/1 -> Divide2/1
  k1/1 -> Product4/3
  Ncs1/1 -> Product4/1
  Divide/1 -> Math Function/1
  Vd/1 -> Divide/1
  1/1 -> Subtract/2
  Math Function/1 -> Subtract/1
  Product1/1 -> Id/1
  [Io] -> Product1/1
  Isc/1 -> Subtract2/1
  Voc/1 -> Subtract5/1
  Subtract6/1 -> Divide4/3
  Subtract2/1 -> Divide4/2
  Np2/1 -> Divide4/1
  Subtract/1 -> Product1/2
  Subtract5/1 -> Divide3/1
  Product7/1 -> Divide3/2
  Tc/1 -> [Tc]
  Ns/1 -> Product2/3

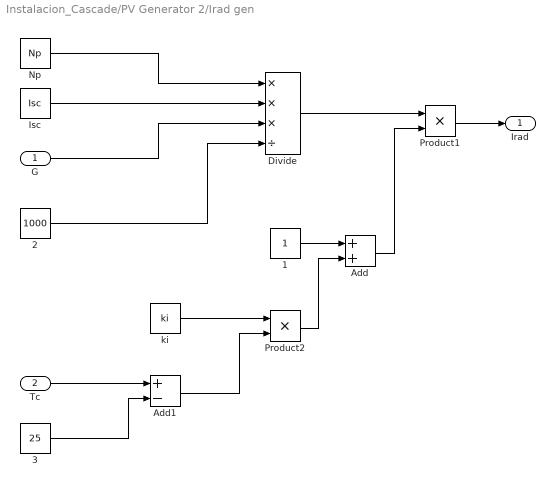
== system Instalacion_Cascade/PV Generator 2/Irad gen ==
  G : Inport
  Tc : Inport  Port=2
  1 : Constant
  2 : Constant  Value=1000
  3 : Constant  Value=25
  Add : Sum
  Add1 : Sum  Inputs=+-
  Divide : Product  Inputs=***/
  Isc : Constant  Value=Isc
  Np : Constant  Value=Np
  Product1 : Product
  Product2 : Product
  ki : Constant  Value=ki
  Irad : Outport
  wires:
  2/1 -> Divide/4
  G/1 -> Divide/3
  Isc/1 -> Divide/2
  Np/1 -> Divide/1
  Divide/1 -> Product1/1
  ki/1 -> Product2/1
  1/1 -> Add/1
  Add/1 -> Product1/2
  Product2/1 -> Add/2
  Tc/1 -> Add1/1
  Add1/1 -> Product2/2
  3/1 -> Add1/2
  Product1/1 -> Irad/1

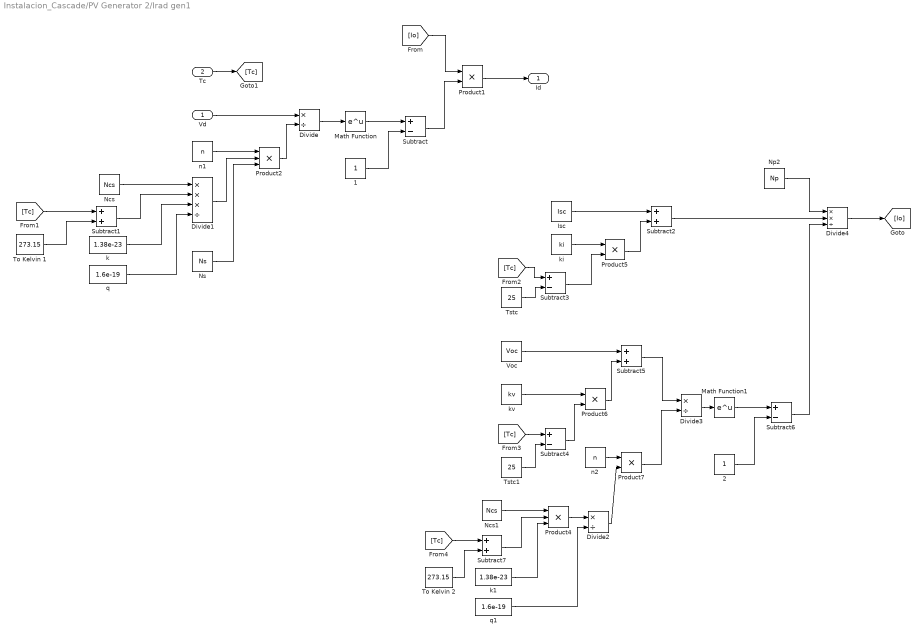
== system Instalacion_Cascade/PV Generator 2/Irad gen1 ==
  Vd : Inport
  Tc : Inport  Port=2
  1 : Constant
  2 : Constant
  Divide : Product  Inputs=*/
  Divide1 : Product  Inputs=***/
  Divide2 : Product  Inputs=*/
  Divide3 : Product  Inputs=*/
  Divide4 : Product  Inputs=**/
  Isc : Constant  Value=Isc
  Math Function : Math  SaturateOnIntegerOverflow=on
  Math Function1 : Math  SaturateOnIntegerOverflow=on
  Ncs : Constant  Value=Ncs
  Ncs1 : Constant  Value=Ncs
  Np2 : Constant  Value=Np
  Ns : Constant  Value=Ns
  Product{1,5..7} (4 alike) : Product
  Product2 : Product  Inputs=3
  Product4 : Product  Inputs=3
  Subtract{,3..4,6} (4 alike) : Sum  Inputs=+-
  Subtract{1..2,5,7} (4 alike) : Sum
  To Kelvin 1 : Constant  Value=273.15
  To Kelvin 2 : Constant  Value=273.15
  Tstc : Constant  Value=25
  Tstc1 : Constant  Value=25
  Voc : Constant  Value=Voc
  k : Constant  Value=1.38e-23
  k1 : Constant  Value=1.38e-23
  ki : Constant  Value=ki
  kv : Constant  Value=kv
  n1 : Constant  Value=n
  n2 : Constant  Value=n
  q : Constant  Value=1.6e-19
  q1 : Constant  Value=1.6e-19
  Id : Outport
  wires:
  Ns/1 -> Product2/3
  Tc/1 -> [Tc]
  Product7/1 -> Divide3/2
  Subtract5/1 -> Divide3/1
  Subtract/1 -> Product1/2
  Np2/1 -> Divide4/1
  Subtract2/1 -> Divide4/2
  Subtract6/1 -> Divide4/3
  Voc/1 -> Subtract5/1
  Isc/1 -> Subtract2/1
  [Io] -> Product1/1
  Product1/1 -> Id/1
  Math Function/1 -> Subtract/1
  1/1 -> Subtract/2
  Vd/1 -> Divide/1
  Divide/1 -> Math Function/1
  Ncs1/1 -> Product4/1
  k1/1 -> Product4/3
  Product4/1 -> Divide2/1
  q1/1 -> Divide2/2
  Divide2/1 -> Product7/2
  ki/1 -> Product5/1
  Product5/1 -> Subtract2/2
  [Tc] -> Subtract3/1
  Tstc/1 -> Subtract3/2
  Subtract3/1 -> Product5/2
  [Tc] -> Subtract4/1
  Tstc1/1 -> Subtract4/2
  kv/1 -> Product6/1
  Subtract4/1 -> Product6/2
  n2/1 -> Product7/1
  Product6/1 -> Subtract5/2
  Divide3/1 -> Math Function1/1
  2/1 -> Subtract6/2
  Math Function1/1 -> Subtract6/1
  Divide4/1 -> [Io]
  Product2/1 -> Divide/2
  n1/1 -> Product2/1
  Divide1/1 -> Product2/2
  Ncs/1 -> Divide1/1
  k/1 -> Divide1/3
  q/1 -> Divide1/4
  Subtract1/1 -> Divide1/2
  [Tc] -> Subtract1/1
  To Kelvin 1/1 -> Subtract1/2
  [Tc] -> Subtract7/1
  Subtract7/1 -> Product4/2
  To Kelvin 2/1 -> Subtract7/2
